simulink model "Robot_Wheel"  (R2018a)
settings: Solver=VariableStepAuto  StartTime=0.0  StopTime=10.0  RelTol=1e-3
values from neighbouring files (symbols this model uses):
  fv_wheel = 0.0    [Robot_Wheel.sldd]
  M_wheel = 0.2    [Robot_Wheel.sldd]
  mu = 1.0    [Robot_Wheel.sldd]
  R_wheel = 0.06    [Robot_Wheel.sldd]
settings Model: DataDictionary=Robot_Wheel.sldd  Creator=hugo  LastModifiedBy=hugo
settings ModelReferenceCC: ModelReferenceMinAlgLoopOccurrences=on

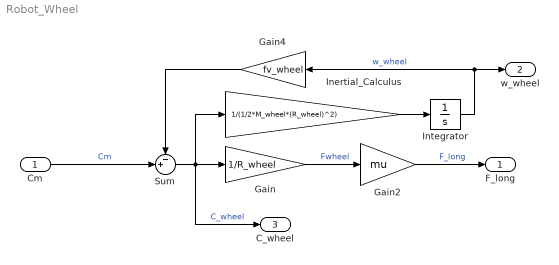
== system Robot_Wheel ==
  Cm : Inport
  Gain : Gain  Gain=1/R_wheel
  Gain2 : Gain  Gain=mu
  Gain4 : Gain  Gain=fv_wheel
  Inertial_Calculus : Gain  Gain=1/(1/2*M_wheel*(R_wheel)^2)
  Integrator : Integrator  ContinuousStateAttributes='w_wheel'
  Sum : Sum  Inputs=-+|
  F_long : Outport
  w_wheel : Outport  Port=2
  C_wheel : Outport  Port=3
  wires:
  Integrator/1 -> Gain4/1, w_wheel/1  "w_wheel"
  Gain/1 -> Gain2/1  "Fwheel"
  Gain4/1 -> Sum/1
  Cm/1 -> Sum/2  "Cm"
  Sum/1 -> C_wheel/1, Inertial_Calculus/1, Gain/1  "C_wheel"
  Gain2/1 -> F_long/1  "F_long"
  Inertial_Calculus/1 -> Integrator/1
